simulink model "Electrical_System_2018b_obfs"  (R2019b)
settings: Solver=VariableStepAuto  StartTime=0.0  StopTime=5  RelTol=1e-3  AbsTol=1e-3  EnableMultiTasking=on
InitFcn:
  | Steady_State_Initialisation;
StopFcn:
  | %sscexplore(simlog);
  | %Logging
undefined symbols (not defined in the file): abrlhklxvp, aexgmhuedq, afmfmjnutg, afpphrjpnc, ahuxbyvruc, alarvljztt, amxnyqmnuw, aodrlwvqie, aolhmuplyq, aqpmguuqkg, auesgwirzl, aurophlnng, awamelrhru, ayfhvxflxn, azxkacuhqc, babszerikg, bawhdqanwq, bevoqecvei, bltjvqbchx, bmqsuewujl, bsmyqjfgnf, btvjbsmnve, bywgxqeadw, bziaduxaer, bzmcmdqocb, bzsvyvetat, ccsjnrbsih, cdvenygxwh, cedkrnslhx, cjheorclzs, cjrdshrtqx, ckhavyhcza, ckxewznhlz, cmrcgyiplk, conenicnws, cqkejbgjnn, csfnuwymhe, cunupkhwbh, cwzfvzuxxh, dcadmadufn, dcfponivnv, ddtrqjrhjn, dfhoxvkqas, dfrhtcwpne, dfvomcagjv, djijwylxea, dnmeqksrrm, dnzewbdkaa, dsqcykyxav, dtswwlttmm, ecumpidjtv, edegaywrct, ejjjsmnejc, eknqnehjdz, emvdetzouf, esxbqkbahr, etnkkbreiq, eunoiiiirw, ewewcuedir, fatkfxdhtc ... (+386)
libraries: fl_lib x802, ee_lib x362, fl_ps_legacy_lib x160, nesl_utility x85
(part 6 of 26)

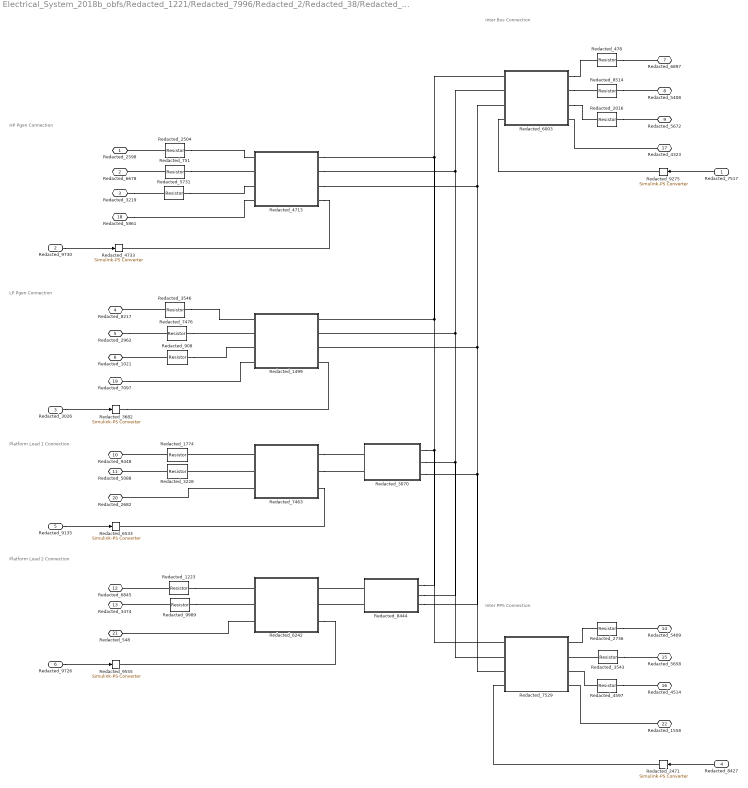
== system Electrical_System_2018b_obfs/Redacted_1221/Redacted_7996/Redacted_2/Redacted_38/Redacted_8107 ==
  note: Platform Load 2 Connection
  note: Platform Load 1 Connection
  note: LP Pgen Connection
  note: HP Pgen Connection
  note: Inter PPS Connection
  note: Inter Bus Connection
  Redacted_7517 : Inport
  Redacted_9730 : Inport  Port=2
  Redacted_3026 : Inport  Port=3
  Redacted_8427 : Inport  Port=4
  Redacted_9135 : Inport  Port=5
  Redacted_9726 : Inport  Port=6
  Redacted_1223 : fl_lib/Electrical/Electrical Elements/Resistor  R=sjdolluzxe Ohm  i_specify=off  i_priority=None  i=ngzdomuwsd A  i_nominal_specify=off  i_nominal_unit=A  i_nominal_value=yvztmdkbhh  v_specify=off  v_priority=None  v=bscchvjlsd V  v_nominal_specify=off  v_nominal_unit=V  v_nominal_value=umzxrcvlku
  Redacted_1499 : Subsystem
      mask Display: image('SSPC.PNG'); % Use "Edit Image" on toolstrip to change.
  Redacted_1774 : fl_lib/Electrical/Electrical Elements/Resistor  R=ubcqenhdwv Ohm  i_specify=off  i_priority=None  i=lonqxilzul A  i_nominal_specify=off  i_nominal_unit=A  i_nominal_value=ngzkpdzjej  v_specify=off  v_priority=None  v=mtbfopdtqe V  v_nominal_specify=off  v_nominal_unit=V  v_nominal_value=ptvlyilmlu
  Redacted_2016 : fl_lib/Electrical/Electrical Elements/Resistor  R=uehuguxvnr Ohm  i_specify=off  i_priority=None  i=gpjoztugsb A  i_nominal_specify=off  i_nominal_unit=A  i_nominal_value=rxdsqmeito  v_specify=off  v_priority=None  v=mnwakbvrrh V  v_nominal_specify=off  v_nominal_unit=V  v_nominal_value=mnwzzbkphc
  Redacted_{2471,3682,4733,6533,9275,9555} (6 alike) : nesl_utility/Simulink-PS Converter  PhysicalDomain=network_engine_domain  SubClassName=ps_input  LeftPortType=input  RightPortType=output  PseudoPeriodic=off  Frequencies=[]  NoiseDistribution=none  NoiseParameters=[]  Unit=1  AffineConversion=off  FilteringAndDerivatives=provide  SimscapeFilterOrder=1  InputFilterTimeConstant=0.001  UdotUserProvided=0
  Redacted_2504 : fl_lib/Electrical/Electrical Elements/Resistor  R=awamelrhru Ohm  i_specify=off  i_priority=None  i=jnkfqgbyzv A  i_nominal_specify=off  i_nominal_unit=A  i_nominal_value=wkfpneyenj  v_specify=off  v_priority=None  v=rkhvctzjlt V  v_nominal_specify=off  v_nominal_unit=V  v_nominal_value=geiusuemea
  Redacted_2736 : fl_lib/Electrical/Electrical Elements/Resistor  R=ldsrjulotb Ohm  i_specify=off  i_priority=None  i=fblccdseua A  i_nominal_specify=off  i_nominal_unit=A  i_nominal_value=oeznhcqnka  v_specify=off  v_priority=None  v=npybdlghir V  v_nominal_specify=off  v_nominal_unit=V  v_nominal_value=gvfezcdtcn
  Redacted_3070 : Subsystem  VariantControlMode=Label  Variant=on  VariantControl=Variant1  LabelModeActiveChoice=Variant2
      mask Display: image('Rail Connection.png'); % Use "Edit Image" on toolstrip to change.
  Redacted_3228 : fl_lib/Electrical/Electrical Elements/Resistor  R=zdgwlscsrc Ohm  i_specify=off  i_priority=None  i=owjpacpnqo A  i_nominal_specify=off  i_nominal_unit=A  i_nominal_value=wwccxdknar  v_specify=off  v_priority=None  v=ackuqqmfxl V  v_nominal_specify=off  v_nominal_unit=V  v_nominal_value=wedppipphf
  Redacted_3543 : fl_lib/Electrical/Electrical Elements/Resistor  R=mrbtfyrlyp Ohm  i_specify=off  i_priority=None  i=kftbgibtup A  i_nominal_specify=off  i_nominal_unit=A  i_nominal_value=ldmyiogtiz  v_specify=off  v_priority=None  v=nnrgkdedip V  v_nominal_specify=off  v_nominal_unit=V  v_nominal_value=nkbhhfsxzn
  Redacted_3546 : fl_lib/Electrical/Electrical Elements/Resistor  R=jhgtovbypo Ohm  i_specify=off  i_priority=None  i=rlpegfrkjz A  i_nominal_specify=off  i_nominal_unit=A  i_nominal_value=oucwhhfkii  v_specify=off  v_priority=None  v=dysxsxinag V  v_nominal_specify=off  v_nominal_unit=V  v_nominal_value=uigskimzev
  Redacted_4597 : fl_lib/Electrical/Electrical Elements/Resistor  R=fvgznnouho Ohm  i_specify=off  i_priority=None  i=jphgmyadjd A  i_nominal_specify=off  i_nominal_unit=A  i_nominal_value=jndactudyu  v_specify=off  v_priority=None  v=lvpeuohgzz V  v_nominal_specify=off  v_nominal_unit=V  v_nominal_value=khxlxscugk
  Redacted_4713 : Subsystem
      mask Display: image('SSPC.PNG'); % Use "Edit Image" on toolstrip to change.
  Redacted_478 : fl_lib/Electrical/Electrical Elements/Resistor  R=hwfgewajfq Ohm  i_specify=off  i_priority=None  i=daiysladyz A  i_nominal_specify=off  i_nominal_unit=A  i_nominal_value=jmtrontctb  v_specify=off  v_priority=None  v=nojnagyxex V  v_nominal_specify=off  v_nominal_unit=V  v_nominal_value=ottkagceil
  Redacted_5731 : fl_lib/Electrical/Electrical Elements/Resistor  R=spitgjqwde Ohm  i_specify=off  i_priority=None  i=klwkvrfgdz A  i_nominal_specify=off  i_nominal_unit=A  i_nominal_value=waiewvjyul  v_specify=off  v_priority=None  v=itobauojdc V  v_nominal_specify=off  v_nominal_unit=V  v_nominal_value=nihyjnollp
  Redacted_6003 : Subsystem
      mask Display: image('SSPC.PNG'); % Use "Edit Image" on toolstrip to change.
  Redacted_6242 : Subsystem
      mask Display: image('SSPC.PNG'); % Use "Edit Image" on toolstrip to change.
  Redacted_7463 : Subsystem
      mask Display: image('SSPC.PNG'); % Use "Edit Image" on toolstrip to change.
  Redacted_7476 : fl_lib/Electrical/Electrical Elements/Resistor  R=gldcydwjeb Ohm  i_specify=off  i_priority=None  i=hjdgndgkrl A  i_nominal_specify=off  i_nominal_unit=A  i_nominal_value=eutsapefwf  v_specify=off  v_priority=None  v=resgdhqgwk V  v_nominal_specify=off  v_nominal_unit=V  v_nominal_value=uxmfwrhjba
  Redacted_751 : fl_lib/Electrical/Electrical Elements/Resistor  R=vvqvpmkxck Ohm  i_specify=off  i_priority=None  i=qbvnbydwpr A  i_nominal_specify=off  i_nominal_unit=A  i_nominal_value=fgrbwwnblb  v_specify=off  v_priority=None  v=wwcilqkvbu V  v_nominal_specify=off  v_nominal_unit=V  v_nominal_value=webjysbuft
  Redacted_7529 : Subsystem
      mask Display: image('SSPC.PNG'); % Use "Edit Image" on toolstrip to change.
  Redacted_8444 : Subsystem  VariantControlMode=Label  Variant=on  VariantControl=Variant1  LabelModeActiveChoice=Variant2
      mask Display: image('Rail Connection.png'); % Use "Edit Image" on toolstrip to change.
  Redacted_8514 : fl_lib/Electrical/Electrical Elements/Resistor  R=vfokesdqjr Ohm  i_specify=off  i_priority=None  i=owrhiolwzf A  i_nominal_specify=off  i_nominal_unit=A  i_nominal_value=lkozpfoafa  v_specify=off  v_priority=None  v=jqwzgqdxiv V  v_nominal_specify=off  v_nominal_unit=V  v_nominal_value=evvjvghatg
  Redacted_908 : fl_lib/Electrical/Electrical Elements/Resistor  R=bevoqecvei Ohm  i_specify=off  i_priority=None  i=jwlzzorzba A  i_nominal_specify=off  i_nominal_unit=A  i_nominal_value=rvqzfkktzi  v_specify=off  v_priority=None  v=bhosuphvek V  v_nominal_specify=off  v_nominal_unit=V  v_nominal_value=qozacnamyt
  Redacted_9989 : fl_lib/Electrical/Electrical Elements/Resistor  R=qrptpvdzui Ohm  i_specify=off  i_priority=None  i=aqwocztkwk A  i_nominal_specify=off  i_nominal_unit=A  i_nominal_value=pywwtpvidk  v_specify=off  v_priority=None  v=pgjzjpdwqq V  v_nominal_specify=off  v_nominal_unit=V  v_nominal_value=pfbusjnjhw
  Redacted_2598 : PMIOPort  Side=Left
  Redacted_6678 : PMIOPort  Port=2  Side=Left
  Redacted_3219 : PMIOPort  Port=3  Side=Left
  Redacted_8217 : PMIOPort  Port=4  Side=Left
  Redacted_2962 : PMIOPort  Port=5  Side=Left
  Redacted_1021 : PMIOPort  Port=6  Side=Left
  Redacted_6897 : PMIOPort  Port=7  Side=Right
  Redacted_5408 : PMIOPort  Port=8  Side=Right
  Redacted_5672 : PMIOPort  Port=9  Side=Right
  Redacted_9448 : PMIOPort  Port=10  Side=Left
  Redacted_5088 : PMIOPort  Port=11  Side=Left
  Redacted_6845 : PMIOPort  Port=12  Side=Left
  Redacted_3474 : PMIOPort  Port=13  Side=Left
  Redacted_5409 : PMIOPort  Port=14  Side=Right
  Redacted_5658 : PMIOPort  Port=15  Side=Right
  Redacted_4514 : PMIOPort  Port=16  Side=Right
  Redacted_4323 : PMIOPort  Port=17  Side=Left
  Redacted_5861 : PMIOPort  Port=18  Side=Left
  Redacted_7097 : PMIOPort  Port=19  Side=Left
  Redacted_2682 : PMIOPort  Port=20  Side=Left
  Redacted_548 : PMIOPort  Port=21  Side=Left
  Redacted_1558 : PMIOPort  Port=22  Side=Left
  wires:
  Redacted_9730/1 -> Redacted_4733/1
  Redacted_3026/1 -> Redacted_3682/1
  Redacted_7517/1 -> Redacted_9275/1
  Redacted_8427/1 -> Redacted_2471/1
  Redacted_9135/1 -> Redacted_6533/1
  Redacted_9726/1 -> Redacted_9555/1
  connections:
  Redacted_4323/RConn1 -- Redacted_6003/LConn4
  Redacted_1558/RConn1 -- Redacted_7529/LConn4
  Redacted_5861/RConn1 -- Redacted_4713/LConn4
  Redacted_7097/RConn1 -- Redacted_1499/LConn4
  Redacted_7463/LConn2 -- Redacted_3228/RConn1
  Redacted_7463/LConn1 -- Redacted_1774/LConn1
  Redacted_6242/RConn3 -- Redacted_9555/RConn1
  Redacted_6242/LConn3 -- Redacted_548/RConn1
  Redacted_8444/RConn2 -- Redacted_6242/RConn2
  Redacted_9989/RConn1 -- Redacted_6242/LConn2
  Redacted_8444/RConn1 -- Redacted_6242/RConn1
  Redacted_1223/LConn1 -- Redacted_6242/LConn1
  Redacted_7463/LConn3 -- Redacted_2682/RConn1
  Redacted_908/RConn1 -- Redacted_1021/RConn1
  Redacted_2962/RConn1 -- Redacted_7476/RConn1
  Redacted_3546/RConn1 -- Redacted_8217/RConn1
  Redacted_6003/LConn1 -- Redacted_478/LConn1
  Redacted_6003/LConn2 -- Redacted_8514/LConn1
  Redacted_6003/LConn3 -- Redacted_2016/LConn1
  Redacted_2016/RConn1 -- Redacted_5672/RConn1
  Redacted_8514/RConn1 -- Redacted_5408/RConn1
  Redacted_478/RConn1 -- Redacted_6897/RConn1
  Redacted_2736/RConn1 -- Redacted_5409/RConn1
  Redacted_3543/RConn1 -- Redacted_5658/RConn1
  Redacted_4597/RConn1 -- Redacted_4514/RConn1
  Redacted_4597/LConn1 -- Redacted_7529/LConn3
  Redacted_3543/LConn1 -- Redacted_7529/LConn2
  Redacted_2736/LConn1 -- Redacted_7529/LConn1
  Redacted_3219/RConn1 -- Redacted_5731/RConn1
  Redacted_751/LConn1 -- Redacted_4713/LConn2
  Redacted_2504/LConn1 -- Redacted_4713/LConn1
  Redacted_3228/LConn1 -- Redacted_5088/RConn1
  Redacted_1223/RConn1 -- Redacted_6845/RConn1
  Redacted_9989/LConn1 -- Redacted_3474/RConn1
  Redacted_6003/RConn3 -- Redacted_1499/RConn3 -- Redacted_3070/LConn3 -- Redacted_8444/LConn3 -- Redacted_7529/RConn3 -- Redacted_4713/RConn3
  Redacted_2504/RConn1 -- Redacted_2598/RConn1
  Redacted_1774/RConn1 -- Redacted_9448/RConn1
  Redacted_3682/RConn1 -- Redacted_1499/RConn4
  Redacted_4713/RConn4 -- Redacted_4733/RConn1
  Redacted_6003/RConn4 -- Redacted_9275/RConn1
  Redacted_2471/RConn1 -- Redacted_7529/RConn4
  Redacted_7463/RConn3 -- Redacted_6533/RConn1
  Redacted_3546/LConn1 -- Redacted_1499/LConn1
  Redacted_7476/LConn1 -- Redacted_1499/LConn2
  Redacted_908/LConn1 -- Redacted_1499/LConn3
  Redacted_751/RConn1 -- Redacted_6678/RConn1
  Redacted_5731/LConn1 -- Redacted_4713/LConn3
  Redacted_6003/RConn1 -- Redacted_1499/RConn1 -- Redacted_3070/LConn1 -- Redacted_8444/LConn1 -- Redacted_7529/RConn1 -- Redacted_4713/RConn1
  Redacted_6003/RConn2 -- Redacted_1499/RConn2 -- Redacted_3070/LConn2 -- Redacted_8444/LConn2 -- Redacted_7529/RConn2 -- Redacted_4713/RConn2
  Redacted_7463/RConn1 -- Redacted_3070/RConn1
  Redacted_7463/RConn2 -- Redacted_3070/RConn2
